simulink model "Control_try_final_2020b"  (R2020b)
settings: Solver=VariableStepAuto  StartTime=0.0  StopTime=inf  RelTol=1e-3
undefined symbols (not defined in the file or in its folder): DiscIntNeverNeededParam
libraries: mobileRoboticsLib x25
(part 5 of 7)

== system Control_try_final_2020b/Team_1_behaviour/T1R3 (defender 1)/Team 1 Behaviour1/min_Distance_Finder/Distance1 ==
  R_1_loc : Inport
  R_3_loc : Inport  Port=2
  Demux : Demux  Outputs=3
  Demux1 : Demux  Outputs=3
  Square : Math  Operator=square  SaturateOnIntegerOverflow=on
  Square Root : Sqrt  SaturateOnIntegerOverflow=on
  Square1 : Math  Operator=square  SaturateOnIntegerOverflow=on
  Sum : Sum  Inputs=|+-
  Sum1 : Sum  Inputs=|+-
  Sum2 : Sum  Inputs=|++
  R1_R3_dis : Outport
  wires:
  Square1/1 -> Sum2/2
  Demux/2 -> Sum1/1
  Sum2/1 -> Square Root/1
  Square/1 -> Sum2/1
  Demux/1 -> Sum/1
  Sum1/1 -> Square1/1
  Demux1/2 -> Sum1/2
  Sum/1 -> Square/1
  Demux1/1 -> Sum/2
  R_1_loc/1 -> Demux/1
  R_3_loc/1 -> Demux1/1
  Square Root/1 -> R1_R3_dis/1

== system Control_try_final_2020b/Team_1_behaviour/T1R3 (defender 1)/Team 1 Behaviour1/min_Distance_Finder/Distance2 ==
  R_1_loc : Inport
  R_4_loc : Inport  Port=2
  Demux : Demux  Outputs=3
  Demux1 : Demux  Outputs=3
  Square : Math  Operator=square  SaturateOnIntegerOverflow=on
  Square Root : Sqrt  SaturateOnIntegerOverflow=on
  Square1 : Math  Operator=square  SaturateOnIntegerOverflow=on
  Sum : Sum  Inputs=|+-
  Sum1 : Sum  Inputs=|+-
  Sum2 : Sum  Inputs=|++
  R1_R4_dis : Outport
  wires:
  Square1/1 -> Sum2/2
  Demux/2 -> Sum1/1
  Sum2/1 -> Square Root/1
  Square/1 -> Sum2/1
  Demux/1 -> Sum/1
  Sum1/1 -> Square1/1
  Demux1/2 -> Sum1/2
  Sum/1 -> Square/1
  Demux1/1 -> Sum/2
  R_1_loc/1 -> Demux/1
  R_4_loc/1 -> Demux1/1
  Square Root/1 -> R1_R4_dis/1

== system Control_try_final_2020b/Team_1_behaviour/T1R3 (defender 1)/Team 1 Behaviour1/min_Distance_Finder/R2_O_dist_val ==
  R_1_loc : Inport
  R_2_loc : Inport  Port=2
  sen_1_val : Inport  Port=3
  Chart : Stateflow chart  TreatAsAtomicUnit=on
  y : Outport
  wires:
  sen_1_val/1 -> Chart/2(sen_1_val)
  R_1_loc/1 -> Chart/1(R_1_loc)
  R_2_loc/1 -> Chart/3(R_2_loc)
  Chart/1(dist) -> y/1

== system Control_try_final_2020b/Team_1_behaviour/T1R3 (defender 1)/Team 1 Behaviour1/min_Distance_Finder/R3_O_dist_val ==
  R_1_loc : Inport
  R_2_loc : Inport  Port=2
  sen_1_val : Inport  Port=3
  Chart : Stateflow chart  TreatAsAtomicUnit=on
  y : Outport
  wires:
  Chart/1(dist) -> y/1
  R_2_loc/1 -> Chart/3(R_2_loc)
  R_1_loc/1 -> Chart/1(R_1_loc)
  sen_1_val/1 -> Chart/2(sen_1_val)

== system Control_try_final_2020b/Team_1_behaviour/T1R3 (defender 1)/Team 1 Behaviour1/min_Distance_Finder/R4_O_dist_val ==
  R_1_loc : Inport
  R_2_loc : Inport  Port=2
  sen_1_val : Inport  Port=3
  Chart : Stateflow chart  TreatAsAtomicUnit=on
  y : Outport
  wires:
  sen_1_val/1 -> Chart/2(sen_1_val)
  R_1_loc/1 -> Chart/1(R_1_loc)
  R_2_loc/1 -> Chart/3(R_2_loc)
  Chart/1(dist) -> y/1

== system Control_try_final_2020b/Team_2_Behaviour/T2_R2(defender)/Team 1 Behaviour1/Subsystem/If Action Subsystem ==
  In1 : Inport
  Action Port : ActionPort  ActionPortLabel=if(u1 > 0)
  Out1 : Outport
  wires:
  In1/1 -> Out1/1

== system Control_try_final_2020b/Team_2_Behaviour/T2_R2(defender)/Team 1 Behaviour1/Subsystem/If Action Subsystem1 ==
  In1 : Inport
  Action Port : ActionPort  ActionPortLabel=else
  Out1 : Outport
  wires:
  In1/1 -> Out1/1

== system Control_try_final_2020b/Team_2_Behaviour/T2_R2(defender)/Team 1 Behaviour1/Subsystem1/If Action Subsystem ==
  In1 : Inport
  Action Port : ActionPort  ActionPortLabel=if(u1 < 5.5)
  reset_pos : Outport
  wires:
  In1/1 -> reset_pos/1

== system Control_try_final_2020b/Team_2_Behaviour/T2_R2(defender)/Team 1 Behaviour1/Subsystem1/If Action Subsystem1 ==
  In1 : Inport
  Action Port : ActionPort  ActionPortLabel=else
  reset_pos : Outport
  wires:
  In1/1 -> reset_pos/1

== system Control_try_final_2020b/Team_2_Behaviour/T2_R2(defender)/Team 1 Behaviour1/Subsystem2/If Action Subsystem ==
  In1 : Inport
  Action Port : ActionPort  ActionPortLabel=if(u1 < 5.5)
  reset_pos : Outport
  wires:
  In1/1 -> reset_pos/1

== system Control_try_final_2020b/Team_2_Behaviour/T2_R2(defender)/Team 1 Behaviour1/Subsystem2/If Action Subsystem1 ==
  In1 : Inport
  Action Port : ActionPort  ActionPortLabel=else
  reset_pos : Outport
  wires:
  In1/1 -> reset_pos/1

== system Control_try_final_2020b/Team_2_Behaviour/T2_R2(defender)/Team 1 Behaviour1/kick_direction1/Angle Finder1 ==
  In1 : Inport
  Abs : Abs
  Atan : Trigonometry  Operator=atan
  Demux : Demux  Outputs=2
  Divide : Product  Inputs=/*
  angle : Outport
  wires:
  Divide/1 -> Atan/1
  Demux/2 -> Divide/2
  Demux/1 -> Divide/1
  Atan/1 -> Abs/1
  Abs/1 -> angle/1
  In1/1 -> Demux/1

== system Control_try_final_2020b/Team_2_Behaviour/T2_R2(defender)/Team 1 Behaviour1/min_Distance_Finder/Distance1 ==
  R_1_loc : Inport
  R_3_loc : Inport  Port=2
  Demux : Demux  Outputs=3
  Demux1 : Demux  Outputs=3
  Square : Math  Operator=square  SaturateOnIntegerOverflow=on
  Square Root : Sqrt  SaturateOnIntegerOverflow=on
  Square1 : Math  Operator=square  SaturateOnIntegerOverflow=on
  Sum : Sum  Inputs=|+-
  Sum1 : Sum  Inputs=|+-
  Sum2 : Sum  Inputs=|++
  R1_R3_dis : Outport
  wires:
  Square1/1 -> Sum2/2
  Demux/2 -> Sum1/1
  Sum2/1 -> Square Root/1
  Square/1 -> Sum2/1
  Demux/1 -> Sum/1
  Sum1/1 -> Square1/1
  Demux1/2 -> Sum1/2
  Sum/1 -> Square/1
  Demux1/1 -> Sum/2
  R_1_loc/1 -> Demux/1
  R_3_loc/1 -> Demux1/1
  Square Root/1 -> R1_R3_dis/1

== system Control_try_final_2020b/Team_2_Behaviour/T2_R2(defender)/Team 1 Behaviour1/min_Distance_Finder/Distance2 ==
  R_1_loc : Inport
  R_4_loc : Inport  Port=2
  Demux : Demux  Outputs=3
  Demux1 : Demux  Outputs=3
  Square : Math  Operator=square  SaturateOnIntegerOverflow=on
  Square Root : Sqrt  SaturateOnIntegerOverflow=on
  Square1 : Math  Operator=square  SaturateOnIntegerOverflow=on
  Sum : Sum  Inputs=|+-
  Sum1 : Sum  Inputs=|+-
  Sum2 : Sum  Inputs=|++
  R1_R4_dis : Outport
  wires:
  Square1/1 -> Sum2/2
  Demux/2 -> Sum1/1
  Sum2/1 -> Square Root/1
  Square/1 -> Sum2/1
  Demux/1 -> Sum/1
  Sum1/1 -> Square1/1
  Demux1/2 -> Sum1/2
  Sum/1 -> Square/1
  Demux1/1 -> Sum/2
  R_1_loc/1 -> Demux/1
  R_4_loc/1 -> Demux1/1
  Square Root/1 -> R1_R4_dis/1

== system Control_try_final_2020b/Team_2_Behaviour/T2_R2(defender)/Team 1 Behaviour1/min_Distance_Finder/R2_O_dist_val ==
  R_1_loc : Inport
  R_2_loc : Inport  Port=2
  sen_1_val : Inport  Port=3
  Chart : Stateflow chart  TreatAsAtomicUnit=on
  y : Outport
  wires:
  sen_1_val/1 -> Chart/2(sen_1_val)
  R_1_loc/1 -> Chart/1(R_1_loc)
  R_2_loc/1 -> Chart/3(R_2_loc)
  Chart/1(dist) -> y/1

== system Control_try_final_2020b/Team_2_Behaviour/T2_R2(defender)/Team 1 Behaviour1/min_Distance_Finder/R3_O_dist_val ==
  R_1_loc : Inport
  R_2_loc : Inport  Port=2
  sen_1_val : Inport  Port=3
  Chart : Stateflow chart  TreatAsAtomicUnit=on
  y : Outport
  wires:
  Chart/1(dist) -> y/1
  R_2_loc/1 -> Chart/3(R_2_loc)
  R_1_loc/1 -> Chart/1(R_1_loc)
  sen_1_val/1 -> Chart/2(sen_1_val)

== system Control_try_final_2020b/Team_2_Behaviour/T2_R2(defender)/Team 1 Behaviour1/min_Distance_Finder/R4_O_dist_val ==
  R_1_loc : Inport
  R_2_loc : Inport  Port=2
  sen_1_val : Inport  Port=3
  Chart : Stateflow chart  TreatAsAtomicUnit=on
  y : Outport
  wires:
  sen_1_val/1 -> Chart/2(sen_1_val)
  R_1_loc/1 -> Chart/1(R_1_loc)
  R_2_loc/1 -> Chart/3(R_2_loc)
  Chart/1(dist) -> y/1

== system Control_try_final_2020b/Team_2_Behaviour/T2_R2(defender)/Team 1 Behaviour1/min_Distance_Finder/nearest robot distance ==
  R_1_loc : Inport
  sen_1_val : Inport  Port=2
  Chart : Stateflow chart  TreatAsAtomicUnit=on
  y : Outport
  wires:
  Chart/1(dist) -> y/1
  R_1_loc/1 -> Chart/1(R_1_loc)
  sen_1_val/1 -> Chart/2(sen_1_val)

== system Control_try_final_2020b/Team_2_Behaviour/T2_R3(Attacker 1)/Team 1 Behaviour1/Subsystem/If Action Subsystem ==
  In1 : Inport
  Action Port : ActionPort  ActionPortLabel=if(u1 > 0)
  Out1 : Outport
  wires:
  In1/1 -> Out1/1

== system Control_try_final_2020b/Team_2_Behaviour/T2_R3(Attacker 1)/Team 1 Behaviour1/Subsystem/If Action Subsystem1 ==
  In1 : Inport
  Action Port : ActionPort  ActionPortLabel=else
  Out1 : Outport
  wires:
  In1/1 -> Out1/1

== system Control_try_final_2020b/Team_2_Behaviour/T2_R3(Attacker 1)/Team 1 Behaviour1/Subsystem1/If Action Subsystem ==
  In1 : Inport
  Action Port : ActionPort  ActionPortLabel=if(u1 > 5.5)
  reset_pos : Outport
  wires:
  In1/1 -> reset_pos/1

== system Control_try_final_2020b/Team_2_Behaviour/T2_R3(Attacker 1)/Team 1 Behaviour1/Subsystem1/If Action Subsystem1 ==
  In1 : Inport
  Action Port : ActionPort  ActionPortLabel=else
  reset_pos : Outport
  wires:
  In1/1 -> reset_pos/1

== system Control_try_final_2020b/Team_2_Behaviour/T2_R3(Attacker 1)/Team 1 Behaviour1/kick_direction1/Angle Finder1 ==
  In1 : Inport
  Abs : Abs
  Atan : Trigonometry  Operator=atan
  Demux : Demux  Outputs=2
  Divide : Product  Inputs=/*
  angle : Outport
  wires:
  Divide/1 -> Atan/1
  Demux/2 -> Divide/2
  Demux/1 -> Divide/1
  Atan/1 -> Abs/1
  Abs/1 -> angle/1
  In1/1 -> Demux/1

== system Control_try_final_2020b/Team_2_Behaviour/T2_R3(Attacker 1)/Team 1 Behaviour1/min_Distance_Finder1/Distance1 ==
  R_1_loc : Inport
  R_3_loc : Inport  Port=2
  Demux : Demux  Outputs=3
  Demux1 : Demux  Outputs=3
  Square : Math  Operator=square  SaturateOnIntegerOverflow=on
  Square Root : Sqrt  SaturateOnIntegerOverflow=on
  Square1 : Math  Operator=square  SaturateOnIntegerOverflow=on
  Sum : Sum  Inputs=|+-
  Sum1 : Sum  Inputs=|+-
  Sum2 : Sum  Inputs=|++
  R1_R3_dis : Outport
  wires:
  Square1/1 -> Sum2/2
  Demux/2 -> Sum1/1
  Sum2/1 -> Square Root/1
  Square/1 -> Sum2/1
  Demux/1 -> Sum/1
  Sum1/1 -> Square1/1
  Demux1/2 -> Sum1/2
  Sum/1 -> Square/1
  Demux1/1 -> Sum/2
  R_1_loc/1 -> Demux/1
  R_3_loc/1 -> Demux1/1
  Square Root/1 -> R1_R3_dis/1

== system Control_try_final_2020b/Team_2_Behaviour/T2_R3(Attacker 1)/Team 1 Behaviour1/min_Distance_Finder1/Distance2 ==
  R_1_loc : Inport
  R_4_loc : Inport  Port=2
  Demux : Demux  Outputs=3
  Demux1 : Demux  Outputs=3
  Square : Math  Operator=square  SaturateOnIntegerOverflow=on
  Square Root : Sqrt  SaturateOnIntegerOverflow=on
  Square1 : Math  Operator=square  SaturateOnIntegerOverflow=on
  Sum : Sum  Inputs=|+-
  Sum1 : Sum  Inputs=|+-
  Sum2 : Sum  Inputs=|++
  R1_R4_dis : Outport
  wires:
  Square1/1 -> Sum2/2
  Demux/2 -> Sum1/1
  Sum2/1 -> Square Root/1
  Square/1 -> Sum2/1
  Demux/1 -> Sum/1
  Sum1/1 -> Square1/1
  Demux1/2 -> Sum1/2
  Sum/1 -> Square/1
  Demux1/1 -> Sum/2
  R_1_loc/1 -> Demux/1
  R_4_loc/1 -> Demux1/1
  Square Root/1 -> R1_R4_dis/1

== system Control_try_final_2020b/Team_2_Behaviour/T2_R3(Attacker 1)/Team 1 Behaviour1/min_Distance_Finder1/R2_O_dist_val ==
  R_1_loc : Inport
  R_2_loc : Inport  Port=2
  sen_1_val : Inport  Port=3
  Chart : Stateflow chart  TreatAsAtomicUnit=on
  y : Outport
  wires:
  sen_1_val/1 -> Chart/2(sen_1_val)
  R_1_loc/1 -> Chart/1(R_1_loc)
  R_2_loc/1 -> Chart/3(R_2_loc)
  Chart/1(dist) -> y/1

== system Control_try_final_2020b/Team_2_Behaviour/T2_R3(Attacker 1)/Team 1 Behaviour1/min_Distance_Finder1/R3_O_dist_val ==
  R_1_loc : Inport
  R_2_loc : Inport  Port=2
  sen_1_val : Inport  Port=3
  Chart : Stateflow chart  TreatAsAtomicUnit=on
  y : Outport
  wires:
  Chart/1(dist) -> y/1
  R_2_loc/1 -> Chart/3(R_2_loc)
  R_1_loc/1 -> Chart/1(R_1_loc)
  sen_1_val/1 -> Chart/2(sen_1_val)

== system Control_try_final_2020b/Team_2_Behaviour/T2_R3(Attacker 1)/Team 1 Behaviour1/min_Distance_Finder1/R4_O_dist_val ==
  R_1_loc : Inport
  R_2_loc : Inport  Port=2
  sen_1_val : Inport  Port=3
  Chart : Stateflow chart  TreatAsAtomicUnit=on
  y : Outport
  wires:
  sen_1_val/1 -> Chart/2(sen_1_val)
  R_1_loc/1 -> Chart/1(R_1_loc)
  R_2_loc/1 -> Chart/3(R_2_loc)
  Chart/1(dist) -> y/1

== system Control_try_final_2020b/Team_2_Behaviour/T2_R3(Attacker 1)/Team 1 Behaviour1/min_Distance_Finder1/nearest robot distance ==
  R_1_loc : Inport
  sen_1_val : Inport  Port=2
  Chart : Stateflow chart  TreatAsAtomicUnit=on
  y : Outport
  wires:
  Chart/1(dist) -> y/1
  R_1_loc/1 -> Chart/1(R_1_loc)
  sen_1_val/1 -> Chart/2(sen_1_val)

== system Control_try_final_2020b/Team_2_Behaviour/T3_R4(Attacker 2)/Team 1 Behaviour1/Subsystem3/If Action Subsystem ==
  In1 : Inport
  Action Port : ActionPort  ActionPortLabel=if(u1 > 0)
  Out1 : Outport
  wires:
  In1/1 -> Out1/1

== system Control_try_final_2020b/Team_2_Behaviour/T3_R4(Attacker 2)/Team 1 Behaviour1/Subsystem3/If Action Subsystem1 ==
  In1 : Inport
  Action Port : ActionPort  ActionPortLabel=else
  Out1 : Outport
  wires:
  In1/1 -> Out1/1

== system Control_try_final_2020b/Team_2_Behaviour/T3_R4(Attacker 2)/Team 1 Behaviour1/Subsystem4/If Action Subsystem ==
  In1 : Inport
  Action Port : ActionPort  ActionPortLabel=if(u1 > 5.5)
  reset_pos : Outport
  wires:
  In1/1 -> reset_pos/1

== system Control_try_final_2020b/Team_2_Behaviour/T3_R4(Attacker 2)/Team 1 Behaviour1/Subsystem4/If Action Subsystem1 ==
  In1 : Inport
  Action Port : ActionPort  ActionPortLabel=else
  reset_pos : Outport
  wires:
  In1/1 -> reset_pos/1

== system Control_try_final_2020b/Team_2_Behaviour/T3_R4(Attacker 2)/Team 1 Behaviour1/kick_direction2/Angle Finder1 ==
  In1 : Inport
  Abs : Abs
  Atan : Trigonometry  Operator=atan
  Demux : Demux  Outputs=2
  Divide : Product  Inputs=/*
  angle : Outport
  wires:
  Divide/1 -> Atan/1
  Demux/2 -> Divide/2
  Demux/1 -> Divide/1
  Atan/1 -> Abs/1
  Abs/1 -> angle/1
  In1/1 -> Demux/1

== system Control_try_final_2020b/Team_2_Behaviour/T3_R4(Attacker 2)/Team 1 Behaviour1/min_Distance_Finder1/Distance1 ==
  R_1_loc : Inport
  R_3_loc : Inport  Port=2
  Demux : Demux  Outputs=3
  Demux1 : Demux  Outputs=3
  Square : Math  Operator=square  SaturateOnIntegerOverflow=on
  Square Root : Sqrt  SaturateOnIntegerOverflow=on
  Square1 : Math  Operator=square  SaturateOnIntegerOverflow=on
  Sum : Sum  Inputs=|+-
  Sum1 : Sum  Inputs=|+-
  Sum2 : Sum  Inputs=|++
  R1_R3_dis : Outport
  wires:
  Square1/1 -> Sum2/2
  Demux/2 -> Sum1/1
  Sum2/1 -> Square Root/1
  Square/1 -> Sum2/1
  Demux/1 -> Sum/1
  Sum1/1 -> Square1/1
  Demux1/2 -> Sum1/2
  Sum/1 -> Square/1
  Demux1/1 -> Sum/2
  R_1_loc/1 -> Demux/1
  R_3_loc/1 -> Demux1/1
  Square Root/1 -> R1_R3_dis/1

== system Control_try_final_2020b/Team_2_Behaviour/T3_R4(Attacker 2)/Team 1 Behaviour1/min_Distance_Finder1/Distance2 ==
  R_1_loc : Inport
  R_4_loc : Inport  Port=2
  Demux : Demux  Outputs=3
  Demux1 : Demux  Outputs=3
  Square : Math  Operator=square  SaturateOnIntegerOverflow=on
  Square Root : Sqrt  SaturateOnIntegerOverflow=on
  Square1 : Math  Operator=square  SaturateOnIntegerOverflow=on
  Sum : Sum  Inputs=|+-
  Sum1 : Sum  Inputs=|+-
  Sum2 : Sum  Inputs=|++
  R1_R4_dis : Outport
  wires:
  Square1/1 -> Sum2/2
  Demux/2 -> Sum1/1
  Sum2/1 -> Square Root/1
  Square/1 -> Sum2/1
  Demux/1 -> Sum/1
  Sum1/1 -> Square1/1
  Demux1/2 -> Sum1/2
  Sum/1 -> Square/1
  Demux1/1 -> Sum/2
  R_1_loc/1 -> Demux/1
  R_4_loc/1 -> Demux1/1
  Square Root/1 -> R1_R4_dis/1

== system Control_try_final_2020b/Team_2_Behaviour/T3_R4(Attacker 2)/Team 1 Behaviour1/min_Distance_Finder1/R2_O_dist_val ==
  R_1_loc : Inport
  R_2_loc : Inport  Port=2
  sen_1_val : Inport  Port=3
  Chart : Stateflow chart  TreatAsAtomicUnit=on
  y : Outport
  wires:
  sen_1_val/1 -> Chart/2(sen_1_val)
  R_1_loc/1 -> Chart/1(R_1_loc)
  R_2_loc/1 -> Chart/3(R_2_loc)
  Chart/1(dist) -> y/1

== system Control_try_final_2020b/Team_2_Behaviour/T3_R4(Attacker 2)/Team 1 Behaviour1/min_Distance_Finder1/R3_O_dist_val ==
  R_1_loc : Inport
  R_2_loc : Inport  Port=2
  sen_1_val : Inport  Port=3
  Chart : Stateflow chart  TreatAsAtomicUnit=on
  y : Outport
  wires:
  Chart/1(dist) -> y/1
  R_2_loc/1 -> Chart/3(R_2_loc)
  R_1_loc/1 -> Chart/1(R_1_loc)
  sen_1_val/1 -> Chart/2(sen_1_val)

== system Control_try_final_2020b/Team_2_Behaviour/T3_R4(Attacker 2)/Team 1 Behaviour1/min_Distance_Finder1/R4_O_dist_val ==
  R_1_loc : Inport
  R_2_loc : Inport  Port=2
  sen_1_val : Inport  Port=3
  Chart : Stateflow chart  TreatAsAtomicUnit=on
  y : Outport
  wires:
  sen_1_val/1 -> Chart/2(sen_1_val)
  R_1_loc/1 -> Chart/1(R_1_loc)
  R_2_loc/1 -> Chart/3(R_2_loc)
  Chart/1(dist) -> y/1

== system Control_try_final_2020b/Team_2_Behaviour/T3_R4(Attacker 2)/Team 1 Behaviour1/min_Distance_Finder1/nearest robot distance ==
  R_1_loc : Inport
  sen_1_val : Inport  Port=2
  Chart : Stateflow chart  TreatAsAtomicUnit=on
  y : Outport
  wires:
  Chart/1(dist) -> y/1
  R_1_loc/1 -> Chart/1(R_1_loc)
  sen_1_val/1 -> Chart/2(sen_1_val)

== matlab function Control_try_final_2020b/Team_1_behaviour/T1R3 (defender 1)/Team 1 Behaviour1/min_Distance_Finder/zero_padding ==
  data: u input; y output
function y = pad(u)
% Zero-pads object detections to work with arrays of buses

y = zeros(7,3);
numElems = min(size(u,1),7);
for idx = 1:numElems
   y(idx,1:3) = u(idx,1:3); 
end
end

== stateflow chart Control_try_final_2020b/Enviornment/Chart1 ==
  state P1_kick
    du:
    KF = [p1(1);p1(2);p1(3);p1(4)]
    bot_tag = 1
  state P5_kick
    du:
    KF = [p5(1);p5(2);p5(3);p5(4)]
    bot_tag = 5
  state no_ball_kick
    du:
    KF = [0;0;0;0]
  state P2_kick
    du:
    KF = p2
    bot_tag = 2
  state P6_kick
    du:
    KF = p6
    bot_tag = 6
  state P3_kick
    du:
    KF = p3
    bot_tag = 3
  state P7_kick
    du:
    KF = p7
    bot_tag = 7
  state P4_kick
    du:
    KF = p4
    bot_tag = 4
  state P8_kick
    du:
    KF = p8
    bot_tag = 8
  (default) -> no_ball_kick
  P5_kick -> no_ball_kick : [p5(4) == 0]
  P1_kick -> no_ball_kick : [p1(4) == 0]
  no_ball_kick -> P5_kick [order 5] : [p5(4) == 1]
  no_ball_kick -> P1_kick [order 1] : [p1(4) == 1]
  no_ball_kick -> P2_kick [order 2] : [p2(4) == 1]
  no_ball_kick -> P6_kick [order 6] : [p6(4) == 1]
  P2_kick -> no_ball_kick : [p2(4) == 0]
  P6_kick -> no_ball_kick : [p6(4) == 0]
  P3_kick -> no_ball_kick : [p3(4) == 0]
  P7_kick -> no_ball_kick : [p7(4) == 0]
  no_ball_kick -> P7_kick [order 7] : [p7(4) == 1]
  no_ball_kick -> P3_kick [order 3] : [p3(4) == 1]
  no_ball_kick -> P8_kick [order 8] : [p8(4) == 1]
  no_ball_kick -> P4_kick [order 4] : [p4(4) == 1]
  P4_kick -> no_ball_kick : [p4(4) == 0]
  P8_kick -> no_ball_kick : [p8(4) == 0]
  data: bot_tag output; p1 input; p2 input; p3 input; p4 input; p5 input; p6 input; p7 input; p8 input; KF output

== stateflow chart Control_try_final_2020b/Team_1_behaviour/T1R1(Goal_Keeper)/Ball_in_D/Chart ==
  state second_coordinate
    du:
    actual_angle = -pi +angle + angle_bot;
  state first_coordinate
    du:
    actual_angle = angle_bot - angle;
  state ffourth_coordinate
    du:
    actual_angle = -(2*pi) + angle + angle_bot
  state Third_coordinate
    du:
    actual_angle =-(pi) - angle + angle_bot;
  (default) -> first_coordinate
  first_coordinate -> second_coordinate [order 1] : [ Rx>Bx && Ry<By ]
  second_coordinate -> first_coordinate [order 1] : [ Rx<Bx && Ry<By]
  ffourth_coordinate -> second_coordinate [order 1] : [ Rx>Bx && Ry<By ]
  first_coordinate -> Third_coordinate [order 3] : [ Rx>Bx && Ry>By]
  second_coordinate -> Third_coordinate [order 3] : [ Rx>Bx && Ry>By ]
  Third_coordinate -> second_coordinate [order 1] : [ Rx>Bx && Ry<By ]
  second_coordinate -> ffourth_coordinate [order 2] : [ Rx<Bx && Ry>By ]
  Third_coordinate -> first_coordinate [order 2] : [ Rx<Bx && Ry<By ]
  ffourth_coordinate -> first_coordinate [order 2] : [ Rx<Bx && Ry<By ]
  first_coordinate -> ffourth_coordinate [order 2] : [ Rx<Bx && Ry>By ]
  Third_coordinate -> ffourth_coordinate [order 3] : [ Rx<Bx && Ry>By ]
  ffourth_coordinate -> Third_coordinate [order 3] : [ Rx>Bx && Ry>By]
  data: Bx input; By input; Rx input; Ry input; angle input; actual_angle output; angle_bot input

== stateflow chart Control_try_final_2020b/Team_1_behaviour/T1R1(Goal_Keeper)/Ball_in_D/Chart3 ==
  state stop
    du:
    w = 0;
    v=0.25 * velocity;
  state RCW
    du:
    w = -1*1;
    v=0;
  state RCCW
    du:
    w =1*1;
    v=0;
  (default) -> stop
  stop -> RCCW [order 2] : [after(1,sec) && DT > 0]
  stop -> RCW [order 1] : [after(1,sec) && DT < 0]
  RCW -> stop [order 1] : [DT<= 0.1 && DT>= -0.1]
  RCCW -> stop [order 1] : [DT<= 0.1 && DT>= -0.1]
  RCCW -> RCW [order 2] : [DT>0]
  RCW -> RCCW [order 2] : [DT<0]
  data: velocity input; v output; DT input; w output

== stateflow chart Control_try_final_2020b/Team_1_behaviour/T1R1(Goal_Keeper)/Ball_in_D/Velocity_Decider ==
  state Robot_Far
    du:
    velocity = 1;
    kick = 0;
  state Robot_Close
    du:
    velocity = 0;
    kick = 1;
  (default) -> Robot_Far
  Robot_Far -> Robot_Close : [DBR <= 0.25]
  Robot_Close -> Robot_Far : [DBR > 0.25]
  data: kick output; DBR input; velocity output

== stateflow chart Control_try_final_2020b/Team_2_Behaviour/T2_R3(Attacker 1)/Team 1 Behaviour1/Chart4 ==
  state go_to_ball
    du:
    kick = 0;
    pass_beh = 0;
    if(distance_to_ball < 0.25)
    pass_beh = pass_behaviour_controller(distance_to_goal,nearest_op,nearest_team);
    i = 0;
    else
    velocity = 0.44;
    end
  state avoid
    velocity = -0.44;
  state pass
    du:
    velocity = 0;
    kick = 1;
  state shoot
    du:
    velocity = 0;
    kick = 1;
  state dribble
    du:
    velocity = 0;
    kick = 1;
  (default) -> go_to_ball
  go_to_ball -> avoid [order 4] : [nearest_rob < 0.3 && nearest_rob < 0 ]
  avoid -> go_to_ball : [nearest_rob > 1 || nearest_rob == 0]
  go_to_ball -> pass [order 1] : [pass_beh == 1&& distance_to_ball < 0.25 ]
  dribble -> go_to_ball : [kick == 1]
  go_to_ball -> dribble [order 3] : [pass_beh == 2 && distance_to_ball < 0.25 ]
  pass -> go_to_ball : [kick == 1]
  go_to_ball -> shoot [order 2] : [pass_beh == 3 && distance_to_ball < 0.25 ]
  shoot -> go_to_ball : [kick == 1]
  data: distancetogoal function_input; nearest_oponent_distance function_input; nearest_team_player_distance function_input; pass_behaviour function_output; kick output =0; distance_to_ball input; velocity output; nearest_team input; nearest_op input; distance_to_goal input; pass_beh output =0; i local =1; nearest_rob input
  function pass_behaviour  = pass_behaviour_controller(distancetogoal,nearest_oponent_distance,nearest_team_player_distance):
    | function pass_behaviour  = pass_behaviour_controller(distancetogoal,nearest_oponent_distance,nearest_team_player_distance)
    | %PASS_BEHAVIOR Summary of this function goes here
    | %   Detailed explanation goes here
    | behaviourFuzzyFile= getFISCodeGenerationData('pass_behaviour.fis');
    | b = evalfis(behaviourFuzzyFile,[distancetogoal,nearest_oponent_distance,nearest_team_player_distance]);
    | 
    | if ( b<0.4 )
    | pass_behaviour=1;
    | elseif ( 0.4<=b && b<0.6 )
    | pass_behaviour=2;
    | else
    | pass_behaviour=3;
    | end
    | 
    | end

== stateflow chart Control_try_final_2020b/Team_1_behaviour/T1R1(Goal_Keeper)/Ball_in_D/kick_direction/Chart1 ==
  state x_pos
    du:
    Vx = 1
  state x_neg
    du:
    Vx = -1
  (default) -> x_pos
  x_pos -> x_neg : [x > 0]
  x_neg -> x_pos : [x<1]
  data: Vx output; x input

== stateflow chart Control_try_final_2020b/Team_1_behaviour/T1R1(Goal_Keeper)/Ball_in_D/kick_direction/Chart2 ==
  state y_pos
    du:
    Vy = 1
  state y_neg
    du:
    Vy = -1
  (default) -> y_pos
  y_pos -> y_neg : [y > 0]
  y_neg -> y_pos : [y<1]
  data: y input; Vy output

== stateflow chart Control_try_final_2020b/Team_1_behaviour/T1R3 (Defender 2)/Chart ==
  state reaching_foul
    du:
    velocity_UA = 1;
    dest = [bx;by;0];
  state ball_in_other_half_did_foul
    en:
    if (foul_loc_y>=7)
    dest = [foul_loc_x;foul_loc_y - 1;0];
    elseif(foul_loc_y<=1)
    dest = [foul_loc_x;foul_loc_y + 1;0];
    end
    kick_UA = 1;
    stop = 1;
  state throwing_foul_not_done
    du:
    dest = [bx;by;0];
    kick_UA = 0;
  state ball_in_our_half
    en:
    dest = [5;4;0];
    kick_UA = 1;
  state stop_bot1
    du:
    velocity_UA = 1;
    dest = [bx;by;0];
  state dont_stop_bot1
    du:
    velocity_UA = 1;
    dest = [bx;by;0];
  state throwing_foul_done
    du:
  state init_pos_reached2
    du:
    velocity_UA = 1;
    dest = [bx;by;0];
  state in_play1
    du:
    dest = [bx;by;0];
    kick_UA = 0;
    stop = 0
    velocity_UA = 0;
  state goal1
    en:
    dest = [5;4;0];
    kick_UA = 1;
    if (did_goal == 1)
    stop = 1;
    else
    stop = 0;
    end
  state init_pos_reached1
    du:
  throwing_foul_not_done -> ball_in_our_half [order 2] : [foul_loc_x < 5.5]
  ball_in_other_half_did_foul -> reaching_foul : [R_2_loc(1) < foul_loc_x + 0.25 &&  R_2_loc(1) > foul_loc_x- 0.25 && R_2_loc(2) < foul_loc_y + 1.25 &&  R_2_loc(2) > foul_loc_y - 1.25 && after(3,sec)]
  init_pos_reached1 -> dont_stop_bot1 [order 2] : [stop == 0]
  reaching_foul -> in_play1 : [bx >foul_loc_x + 0.1  || bx < foul_loc_x - 0.1|| by >foul_loc_y + 0.1 || by<foul_loc_y - 0.1]
  throwing_foul_done -> ball_in_other_half_did_foul [order 1] : [foul_loc_x > 5.5]
  in_play1 -> throwing_foul_not_done [order 3] : [foul_team_right == 1]
  throwing_foul_not_done -> in_play1 [order 1] : [foul_loc_x > 5.5 && after(2,sec)]
  init_pos_reached1 -> stop_bot1 [order 1] : [stop == 1]
  throwing_foul_done -> ball_in_our_half [order 2] : [foul_loc_x < 5.5]
  ball_in_our_half -> init_pos_reached2 : [R_2_loc(1) <5.25 &&  R_2_loc(1) >4.75 && R_2_loc(2) <4.25 &&  R_2_loc(2) >3.75 && after(2,sec)]
  in_play1 -> throwing_foul_done [order 2] : [foul_team_left == 1]
  dont_stop_bot1 -> in_play1 : [reset == 0 && after(3,sec)]
  stop_bot1 -> in_play1 : [bx > 5.6 || bx < 5.4 || by >4.1 || by<3.9]
  (default) -> in_play1
  init_pos_reached2 -> in_play1 : [[bx >foul_loc_x + 0.1  || bx < foul_loc_x - 0.1|| by >foul_loc_y + 0.1 || by<foul_loc_y - 0.1]]
  goal1 -> init_pos_reached1 : [R_2_loc(1) <5.25 &&  R_2_loc(1) >4.75 && R_2_loc(2) <4.25 &&  R_2_loc(2) >3.75 && after(3,sec) ]
  in_play1 -> goal1 [order 1] : [reset == 1]
  data: R_2_loc input; bx input; by input; foul_team_right input; foul_team_left input; did_goal input; foul_loc_x input; foul_loc_y input; reset input; dest output; kick_UA output; velocity_UA output; stop local

== stateflow chart Control_try_final_2020b/Team_2_Behaviour/T2_R2(defender)/Chart ==
  state reaching_foul
    du:
    velocity_UA = 1;
    dest = [bx;by;0];
  state ball_in_other_half_did_foul
    en:
    if (foul_loc_y>=7)
    dest = [foul_loc_x;foul_loc_y - 1;0];
    elseif(foul_loc_y<=1)
    dest = [foul_loc_x;foul_loc_y + 1;0];
    end
    kick_UA = 1;
    stop = 1;
  state throwing_foul_done
    du:
  state throwing_foul_not_done
    du:
    dest = [bx;by;0];
    kick_UA = 0;
  state ball_in_our_half
    en:
    dest = [7.25;2.5;0];
    kick_UA = 1;
  state stop_bot1
    du:
    velocity_UA = 1;
    dest = [bx;by;0];
  state dont_stop_bot1
    du:
    velocity_UA = 1;
    dest = [bx;by;0];
  state init_pos_reached2
    du:
    velocity_UA = 1;
    dest = [bx;by;0];
  state in_play1
    du:
    dest = [bx;by;0];
    kick_UA = 0;
    stop = 0
    velocity_UA = 0;
  state goal1
    en:
    dest = [7.25;2.5;0];
    kick_UA = 1;
    if (did_goal == 1)
    stop = 1;
    else
    stop = 0;
    end
  state init_pos_reached1
    du:
  throwing_foul_not_done -> ball_in_our_half [order 2] : [foul_loc_x < 6]
  ball_in_other_half_did_foul -> reaching_foul : [R_2_loc(1) < foul_loc_x + 0.25 &&  R_2_loc(1) > foul_loc_x- 0.25 && R_2_loc(2) < foul_loc_y + 1.25 &&  R_2_loc(2) > foul_loc_y - 1.25 && after(3,sec)]
  reaching_foul -> in_play1 : [bx >foul_loc_x + 0.1  || bx < foul_loc_x - 0.1|| by >foul_loc_y + 0.1 || by<foul_loc_y - 0.1]
  throwing_foul_done -> ball_in_other_half_did_foul [order 1] : [foul_loc_x < 6]
  throwing_foul_done -> ball_in_our_half [order 2] : [foul_loc_x > 6]
  in_play1 -> throwing_foul_done [order 1] : [foul_team_right == 1]
  in_play1 -> throwing_foul_not_done [order 3] : [foul_team_left == 1]
  throwing_foul_not_done -> in_play1 [order 1] : [foul_loc_x > 6 && after(2,sec)]
  init_pos_reached1 -> dont_stop_bot1 [order 2] : [stop == 0]
  ball_in_our_half -> init_pos_reached2 : [R_2_loc(1) <7.5 &&  R_2_loc(1) >7 && R_2_loc(2) <2.75 &&  R_2_loc(2) >2.25 && after(3,sec)]
  init_pos_reached1 -> stop_bot1 [order 1] : [stop == 1]
  dont_stop_bot1 -> in_play1 : [reset == 0 && after(3,sec)]
  stop_bot1 -> in_play1 : [bx > 5.6 || bx < 5.4 || by >4.1 || by<3.9]
  (default) -> in_play1
  init_pos_reached2 -> in_play1 : [[bx >foul_loc_x + 0.1  || bx < foul_loc_x - 0.1|| by >foul_loc_y + 0.1 || by<foul_loc_y - 0.1]]
  goal1 -> init_pos_reached1 : [R_2_loc(1) <7.5 &&  R_2_loc(1) >7 && R_2_loc(2) <2.75 &&  R_2_loc(2) >2.25 && after(3,sec)]
  in_play1 -> goal1 [order 2] : [reset == 1]
  data: R_2_loc input; bx input; by input; foul_loc_x input; foul_loc_y input; foul_team_left input; foul_team_right input; did_goal input; reset input; dest output; kick_UA output; stop local size=1; velocity_UA output

== stateflow chart Control_try_final_2020b/Team_2_Behaviour/T2_R3(Attacker 1)/Chart ==
  state ball_in_other_half_did_foul
    en:
    if (foul_loc_y>=7)
    dest = [foul_loc_x;foul_loc_y - 1;0];
    elseif(foul_loc_y<=1)
    dest = [foul_loc_x;foul_loc_y + 1;0];
    end
    kick_UA = 1;
    stop = 1;
  state reaching_foul
    du:
    velocity_UA = 1;
    dest = [bx;by;0];
  state throwing_foul_not_done
    du:
    dest = [foul_loc_x;foul_loc_y;0];
    kick_UA = 1;
  state throwing_foul_done
    du:
  state ball_in_our_half
    en:
    dest = [7.25;5.5;0];
    kick_UA = 1;
  state stop_bot
    du:
    velocity_UA = 1;
    dest = [bx;by;0];
  state dont_stop_bot
    du:
    velocity_UA = 1;
    dest = [bx;by;0];
  state in_play1
    du:
    dest = [bx;by;0];
    kick_UA = 0;
    stop = 0
    velocity_UA = 0;
  state goal1
    en:
    dest = [7.25;5.5;0];
    kick_UA = 1;
    if (did_goal == 1)
    stop = 1;
    else
    stop = 0;
    end
  state init_pos_reached1
    du:
  state init_pos
    du:
    velocity_UA = 1;
    dest = [bx;by;0];
  throwing_foul_not_done -> ball_in_our_half [order 2] : [foul_loc_x > 6]
  ball_in_other_half_did_foul -> reaching_foul : [R_2_loc(1) < foul_loc_x + 0.25 &&  R_2_loc(1) > foul_loc_x- 0.25 && R_2_loc(2) < foul_loc_y + 1.25 &&  R_2_loc(2) > foul_loc_y - 1.25 && after(3,sec)]
  throwing_foul_done -> ball_in_other_half_did_foul [order 1] : [foul_loc_x < 6]
  reaching_foul -> in_play1 : [bx >foul_loc_x + 0.1  || bx < foul_loc_x - 0.1|| by >foul_loc_y + 0.1 || by<foul_loc_y - 0.1]
  in_play1 -> throwing_foul_not_done [order 3] : [foul_team_left == 1 && after(2,sec)]
  throwing_foul_not_done -> in_play1 [order 1] : [foul_loc_x < 6 && after(20,sec) &&  bx < foul_loc_x + 0.1  && bx > foul_loc_x - 0.1 && by < foul_loc_y + 0.1  && by > foul_loc_y - 0.1]
  init_pos_reached1 -> dont_stop_bot [order 2] : [stop == 0]
  init_pos_reached1 -> stop_bot [order 1] : [stop == 1]
  throwing_foul_done -> ball_in_our_half [order 2] : [foul_loc_x > 6]
  in_play1 -> throwing_foul_done [order 1] : [foul_team_right == 1]
  ball_in_our_half -> init_pos : [R_2_loc(1) <7.5 &&  R_2_loc(1) >7 && R_2_loc(2) <5.75 &&  R_2_loc(2) >5.25 &&after(3,sec)]
  dont_stop_bot -> in_play1 : [reset == 0 && after(3,sec)]
  stop_bot -> in_play1 : [bx > 5.6 || bx < 5.4 || by >4.1 || by<3.9]
  (default) -> in_play1
  goal1 -> init_pos_reached1 : [R_2_loc(1) <7.5 &&  R_2_loc(1) >7 && R_2_loc(2) <5.75 &&  R_2_loc(2) >5.25 &&after(3,sec)]
  in_play1 -> goal1 [order 2] : [reset == 1]
  init_pos -> in_play1 : [[bx >foul_loc_x + 0.1  || bx < foul_loc_x - 0.1|| by >foul_loc_y + 0.1 || by<foul_loc_y - 0.1]]
  data: R_2_loc input; bx input; by input; foul_loc_x input; foul_loc_y input; foul_team_left input; foul_team_right input; did_goal input; reset input; dest output; kick_UA output; velocity_UA output; stop local

== stateflow chart Control_try_final_2020b/Team_2_Behaviour/T3_R4(Attacker 2)/Chart ==
  state ball_in_other_half_did_foul
    en:
    if (foul_loc_y>=7)
    dest = [foul_loc_x;foul_loc_y - 1;0];
    elseif(foul_loc_y<=1)
    dest = [foul_loc_x;foul_loc_y + 1;0];
    end
    kick_UA = 1;
    stop = 1;
  state reaching_foul
    du:
    velocity_UA = 1;
    dest = [bx;by;0];
  state throwing_foul_done
    du:
  state ball_in_our_half
    en:
    dest = [6;4;0];
    kick_UA = 1;
  state init_pos_reached2
    du:
    velocity_UA = 1;
    dest = [bx;by;0];
  state in_play1
    du:
    dest = [bx;by;0];
    kick_UA = 0;
    stop = 0
    velocity_UA = 0;
  state goal1
    en:
    dest = [6;4;0];
    kick_UA = 1;
    if (did_goal == 1)
    stop = 1;
    else
    stop = 0;
    end
  state reach_pos_CF
    en:
    velocity_UA = 1;
    dest = [bx;by;0];
  state Corner_foul_done
    en:
    dest = [3;2;0];
    kick_UA = 1;
  state init_pos_reached1
    du:
  state stop_bot
    du:
    velocity_UA = 1;
    dest = [bx;by;0];
  state dont_stop_bot
    du:
    velocity_UA = 1;
    dest = [bx;by;0];
  state corner_foul_not_done
    en:
    dest = [C_foul_loc_x;C_foul_loc_y;0];
    kick_UA = 1;
  ball_in_other_half_did_foul -> reaching_foul : [R_2_loc(1) < foul_loc_x + 1.25 &&  R_2_loc(1) > foul_loc_x- 1.25 && R_2_loc(2) < foul_loc_y + 1.25 &&  R_2_loc(2) > foul_loc_y - 1.25 && after(3,sec)]
  throwing_foul_done -> ball_in_other_half_did_foul [order 1] : [foul_loc_x < 6]
  reaching_foul -> in_play1 : [bx >foul_loc_x + 0.1  || bx < foul_loc_x - 0.1|| by >foul_loc_y + 0.1 || by<foul_loc_y - 0.1]
  throwing_foul_done -> ball_in_our_half [order 2] : [foul_loc_x > 6]
  in_play1 -> throwing_foul_done [order 1] : [foul_team_right == 1 || foul_team_left == 1 && after(1,sec)]
  ball_in_our_half -> init_pos_reached2 : [R_2_loc(1) <6.25 &&  R_2_loc(1) >5.75 && R_2_loc(2) <4.25 &&  R_2_loc(2) >3.75 && after(3,sec)]
  init_pos_reached2 -> in_play1 : [[bx >foul_loc_x + 0.1  || bx < foul_loc_x - 0.1|| by >foul_loc_y + 0.1 || by<foul_loc_y - 0.1]]
  (default) -> in_play1
  reach_pos_CF -> in_play1 : [(bx >1.6  || bx < 1.4 || by > 4.1 || by<3.9) && after(1,sec)]
  in_play1 -> goal1 [order 2] : [reset == 1]
  in_play1 -> Corner_foul_done [order 3] : [CFR == 1]
  in_play1 -> corner_foul_not_done [order 4] : [CFL == 1 && after(0.5,sec)]
  corner_foul_not_done -> in_play1 : [[R_2_loc(1) < C_foul_loc_x + 0.25 &&  R_2_loc(1) > C_foul_loc_x- 0.25 && R_2_loc(2) < C_foul_loc_y + 1.25 &&  R_2_loc(2) > C_foul_loc_y - 1.25 && after(3,sec)]]
  dont_stop_bot -> in_play1 : [reset == 0 && after(3,sec)]
  stop_bot -> in_play1 : [bx > 5.6 || bx < 5.4 || by >4.1 || by<3.9]
  goal1 -> init_pos_reached1 : [R_2_loc(1) <6.25 &&  R_2_loc(1) >5.75 && R_2_loc(2) <4.25 &&  R_2_loc(2) >3.75 && after(3,sec)]
  Corner_foul_done -> reach_pos_CF : [[(R_2_loc(1) <3.25 &&  R_2_loc(1) >2.75 && R_2_loc(2) <2.25 &&  R_2_loc(2) >1.75) ]]
  init_pos_reached1 -> stop_bot [order 1] : [stop == 1]
  init_pos_reached1 -> dont_stop_bot [order 2] : [stop == 0]
  data: R_2_loc input; bx input; by input; foul_loc_x input; foul_loc_y input; foul_team_left input; foul_team_right input; did_goal input; CFL input; CFR input; C_foul_loc_x input; C_foul_loc_y input; reset input; dest output; kick_UA output; stop local; velocity_UA output

== stateflow chart Control_try_final_2020b/Team_2_Behaviour/T2_R2(defender)/Team 1 Behaviour1/Chart1 ==
  state second_coordinate
    du:
    actual_angle = -pi +angle + angle_bot;
  state first_coordinate
    du:
    actual_angle = angle_bot - angle;
  state ffourth_coordinate
    du:
    actual_angle = -(2*pi) + angle + angle_bot
  state Third_coordinate
    du:
    actual_angle =-(pi) - angle + angle_bot;
  (default) -> first_coordinate
  first_coordinate -> second_coordinate [order 1] : [ Rx>Bx && Ry<By ]
  second_coordinate -> first_coordinate [order 1] : [ Rx<Bx && Ry<By]
  ffourth_coordinate -> second_coordinate [order 1] : [ Rx>Bx && Ry<By ]
  first_coordinate -> Third_coordinate [order 3] : [ Rx>Bx && Ry>By]
  second_coordinate -> Third_coordinate [order 3] : [ Rx>Bx && Ry>By ]
  Third_coordinate -> second_coordinate [order 1] : [ Rx>Bx && Ry<By ]
  second_coordinate -> ffourth_coordinate [order 2] : [ Rx<Bx && Ry>By ]
  Third_coordinate -> first_coordinate [order 2] : [ Rx<Bx && Ry<By ]
  ffourth_coordinate -> first_coordinate [order 2] : [ Rx<Bx && Ry<By ]
  first_coordinate -> ffourth_coordinate [order 2] : [ Rx<Bx && Ry>By ]
  Third_coordinate -> ffourth_coordinate [order 3] : [ Rx<Bx && Ry>By ]
  ffourth_coordinate -> Third_coordinate [order 3] : [ Rx>Bx && Ry>By]
  data: Bx input; By input; Rx input; Ry input; angle input; actual_angle output; angle_bot input

== stateflow chart Control_try_final_2020b/Team_2_Behaviour/T2_R2(defender)/Team 1 Behaviour1/Chart2 ==
  state go_to_ball
    du:
    kick = 0;
    pass_beh = 0;
    if(distance_to_ball < 0.25)
    pass_beh = pass_behaviour_controller(distance_to_goal,nearest_op,nearest_team);
    i = 0;
    else
    velocity = 0.44;
    end
  state avoid
    velocity = -(velocity);
  state pass
    du:
    velocity = 0;
    kick = 1;
  state shoot
    du:
    velocity = 0;
    kick = 1;
  state dribble
    du:
    velocity = 0;
    kick = 1;
  (default) -> go_to_ball
  go_to_ball -> avoid [order 1] : [nearest_rob < 0.3 && nearest_rob < 0 ]
  avoid -> go_to_ball : [nearest_rob > 1 ]
  go_to_ball -> pass [order 2] : [pass_beh == 1&& distance_to_ball < 0.25 ]
  dribble -> go_to_ball : [kick == 1]
  go_to_ball -> dribble [order 4] : [pass_beh == 2 && distance_to_ball < 0.25 ]
  pass -> go_to_ball : [kick == 1]
  go_to_ball -> shoot [order 3] : [pass_beh == 3 && distance_to_ball < 0.25 ]
  shoot -> go_to_ball : [kick == 1]
  data: distancetogoal function_input; nearest_oponent_distance function_input; nearest_team_player_distance function_input; pass_behaviour function_output; kick output =0; distance_to_ball input; velocity output; nearest_team input; nearest_op input; distance_to_goal input; pass_beh output =0; i local =1; nearest_rob input
  function pass_behaviour  = pass_behaviour_controller(distancetogoal,nearest_oponent_distance,nearest_team_player_distance):
    | function pass_behaviour  = pass_behaviour_controller(distancetogoal,nearest_oponent_distance,nearest_team_player_distance)
    | %PASS_BEHAVIOR Summary of this function goes here
    | %   Detailed explanation goes here
    | behaviourFuzzyFile= getFISCodeGenerationData('pass_behaviour.fis');
    | b = evalfis(behaviourFuzzyFile,[distancetogoal,nearest_oponent_distance,nearest_team_player_distance]);
    | 
    | if ( b<0.4 )
    | pass_behaviour=1;
    | elseif ( 0.4<=b && b<0.6 )
    | pass_behaviour=2;
    | else
    | pass_behaviour=3;
    | end
    | 
    | end

== stateflow chart Control_try_final_2020b/Team_2_Behaviour/T2_R2(defender)/Team 1 Behaviour1/Chart4 ==
  state stop
    du:
    w = 0;
    v=0.25 * velocity;
  state RCW
    du:
    w = -1*1;
    v=0;
  state RCCW
    du:
    w =1*1;
    v=0;
  (default) -> stop
  stop -> RCCW [order 2] : [after(1,sec) && DT > 0]
  stop -> RCW [order 1] : [after(1,sec) && DT < 0]
  RCW -> stop [order 1] : [DT<= 0.1 && DT>= -0.1]
  RCCW -> stop [order 1] : [DT<= 0.1 && DT>= -0.1]
  RCCW -> RCW [order 2] : [DT>0]
  RCW -> RCCW [order 2] : [DT<0]
  data: velocity input; v output; DT input; w output

== matlab function Control_try_final_2020b/Team_2_Behaviour/T2_R2(defender)/Team 1 Behaviour1/MATLAB Function ==
  data: F input; dF output; dis input; dT input
function dF = fcn(F,dis,dT)


F_x_max = max(abs(F(:,1))) ;
% F_y_max = max(abs(F(:,2))) ;

Fmax = sqrt((F_x_max^2)) ;

fc = sqrt(2*dis*dis*dT) ;

if fc <= Fmax
    dF = fc ;
else
    dF = Fmax ;
end

end

== matlab function Control_try_final_2020b/Team_2_Behaviour/T2_R2(defender)/Team 1 Behaviour1/MATLAB Function1 ==
  data: beh input; y output; goal input; team input; rob_loc input; rob_loc1 input; z output
function [y, z] = fcn(beh,goal,team,rob_loc,rob_loc1)
if (beh == 3)
    y = goal;
    z = [10,4];
elseif (beh == 2)
    y = 0.25;
    z = [10,4];
else
    y = team;
    z = [rob_loc1(1), rob_loc1(2)];
end

== stateflow chart Control_try_final_2020b/Team_1_behaviour/T1R2 (attacker 1)/Chart1 ==
  state reaching_foul
    du:
    velocity_UA = 1;
    dest = [bx;by;0];
  state ball_in_other_half_did_foul
    en:
    if (foul_loc_y>=7)
    dest = [foul_loc_x;foul_loc_y - 1;0];
    elseif(foul_loc_y<=1)
    dest = [foul_loc_x;foul_loc_y + 1;0];
    end
    kick_UA = 1;
    stop = 1;
  state throwing_foul
    du:
  state stop_bot1
    du:
    velocity_UA = 1;
    dest = [bx;by;0];
  state dont_stop_bot1
    du:
    velocity_UA = 1;
    dest = [bx;by;0];
  state ball_in_our_half
    en:
    dest = [3.25;2.5;0];
    kick_UA = 1;
  state init_pos_reached2
    du:
    velocity_UA = 1;
    dest = [bx;by;0];
  state in_play1
    du:
    dest = [bx;by;0];
    kick_UA = 0;
    stop = 0
    velocity_UA = 0;
  state goal1
    en:
    dest = [3.25;2.5;0];
    kick_UA = 1;
    if (did_goal == 1)
    stop = 1;
    else
    stop = 0;
    end
  state init_pos_reached1
    du:
  ball_in_other_half_did_foul -> reaching_foul : [R_2_loc(1) < foul_loc_x + 0.25 &&  R_2_loc(1) > foul_loc_x- 0.25 && R_2_loc(2) < foul_loc_y + 1.25 &&  R_2_loc(2) > foul_loc_y - 1.25 && after(3,sec)]
  reaching_foul -> in_play1 : [bx >foul_loc_x + 0.1  || bx < foul_loc_x - 0.1|| by >foul_loc_y + 0.1 || by<foul_loc_y - 0.1]
  init_pos_reached1 -> dont_stop_bot1 [order 2] : [stop == 0]
  throwing_foul -> ball_in_other_half_did_foul [order 1] : [foul_loc_x < 5.5]
  init_pos_reached1 -> stop_bot1 [order 1] : [stop == 1]
  throwing_foul -> ball_in_our_half [order 2] : [foul_loc_x > 5.5]
  in_play1 -> throwing_foul [order 1] : [foul_team_left == 1 || foul_team_right == 1]
  ball_in_our_half -> init_pos_reached2 : [R_2_loc(1) <3.5 &&  R_2_loc(1) >3 && R_2_loc(2) <2.75 &&  R_2_loc(2) >2.25 && after(3,sec)]
  dont_stop_bot1 -> in_play1 : [reset == 0 && after(3,sec)]
  stop_bot1 -> in_play1 : [bx > 5.6 || bx < 5.4 || by >4.1 || by<3.9]
  (default) -> in_play1
  goal1 -> init_pos_reached1 : [R_2_loc(1) <3.5 &&  R_2_loc(1) >3 && R_2_loc(2) <2.75 &&  R_2_loc(2) >2.25 && after(3,sec)]
  in_play1 -> goal1 [order 2] : [reset == 1]
  init_pos_reached2 -> in_play1 : [[bx >foul_loc_x + 0.1  || bx < foul_loc_x - 0.1|| by >foul_loc_y + 0.1 || by<foul_loc_y - 0.1]]
  data: R_2_loc input; bx input; by input; foul_team_right input; foul_team_left input; foul_loc_x input; foul_loc_y input; reset input; dest output; kick_UA output; velocity_UA output; did_goal input; stop local

== stateflow chart Control_try_final_2020b/Referee/Throwing ==
  state initilize
    en:
    foul_team_right = 0;
    foul_team_left = 0;
    throwin_foul_loc = [0;0]
  state out_filed
    en:
    if(bot_tag <5)
    foul_team_left = 1;
    foul_team_right = 0;
    else
    foul_team_left = 0;
    foul_team_right = 1;
    end
    throwin_foul_loc = [X;Y];
  state in_filed
    en:
    foul_team_right = 0;
    foul_team_left = 0;
    throwin_foul_loc = [0;0];
  (default) -> initilize
  initilize -> in_filed : [Y>=1 && Y<=7]
  in_filed -> out_filed : [Y>7 || Y<1]
  out_filed -> in_filed : [Y>=1 && Y<=7]
  data: foul_team_right output; X input; bot_tag input; Y input; foul_team_left output; throwin_foul_loc output

== matlab function Control_try_final_2020b/Enviornment/Ball_Dynamics1/MATLAB Function ==
  data: bot_tag input; pos input size=[1 3]; flag output
function flag  = fcn(bot_tag, pos)

X = pos(1) ;
Y = pos(2) ;
Z = pos(3) ;

% goal conditions
if X < 1 && Y > 2.7  && Y < 5.3 && Z < 1.2 
    flag = [1,5.5,4] ;
elseif fix(X) == 10 && Y > 2.7  && Y < 5.3 && Z <1.2
    flag = [1,5.5,4] ;
    
%corner conditions
elseif (X < 1 && (Y < 2.7 || Y > 5.3))
    if (bot_tag < 5)
        if (Y > 4)
            flag = [1,1,7] ;
        else
            flag = [1,1,1] ;
        end
    else
        flag = [1,1.5,4];
    end
elseif (X > 10 && (Y < 2.7 || Y > 5.3))
    if (bot_tag > 4)
        if (Y > 4)
             flag = [1,10,7] ;
        else
             flag = [1,10,1] ;
        end
    else
        flag = [1,5.5,4];
    end
% throwing conditions
elseif (Y < 1 || Y > 7)
     flag = [1,X,Y] ; 
% in game conditions
else
    flag = [0,5.5,4] ;
end

end

== stateflow chart Control_try_final_2020b/Team_1_behaviour/T1R2 (attacker 1)/Team 1 Behaviour1/Chart1 ==
  state second_coordinate
    du:
    actual_angle = -pi +angle + angle_bot;
  state first_coordinate
    du:
    actual_angle = angle_bot - angle;
  state ffourth_coordinate
    du:
    actual_angle = -(2*pi) + angle + angle_bot
  state Third_coordinate
    du:
    actual_angle =-(pi) - angle + angle_bot;
  (default) -> first_coordinate
  first_coordinate -> second_coordinate [order 1] : [ Rx>Bx && Ry<By ]
  second_coordinate -> first_coordinate [order 1] : [ Rx<Bx && Ry<By]
  ffourth_coordinate -> second_coordinate [order 1] : [ Rx>Bx && Ry<By ]
  first_coordinate -> Third_coordinate [order 3] : [ Rx>Bx && Ry>By]
  second_coordinate -> Third_coordinate [order 3] : [ Rx>Bx && Ry>By ]
  Third_coordinate -> second_coordinate [order 1] : [ Rx>Bx && Ry<By ]
  second_coordinate -> ffourth_coordinate [order 2] : [ Rx<Bx && Ry>By ]
  Third_coordinate -> first_coordinate [order 2] : [ Rx<Bx && Ry<By ]
  ffourth_coordinate -> first_coordinate [order 2] : [ Rx<Bx && Ry<By ]
  first_coordinate -> ffourth_coordinate [order 2] : [ Rx<Bx && Ry>By ]
  Third_coordinate -> ffourth_coordinate [order 3] : [ Rx<Bx && Ry>By ]
  ffourth_coordinate -> Third_coordinate [order 3] : [ Rx>Bx && Ry>By]
  data: Bx input; By input; Rx input; Ry input; angle input; actual_angle output; angle_bot input

== stateflow chart Control_try_final_2020b/Team_1_behaviour/T1R2 (attacker 1)/Team 1 Behaviour1/Chart2 ==
  state go_to_ball
    du:
    kick = 0;
    pass_beh = 0;
    if(distance_to_ball < 0.25)
    pass_beh = pass_behaviour_controller(distance_to_goal,nearest_op,nearest_team);
    i = 0;
    else
    velocity = 0.44;
    end
  state pass
    du:
    velocity = 0;
    kick = 1;
  state shoot
    du:
    velocity = 0;
    kick = 1;
  state dribble
    du:
    velocity = 0;
    kick = 1;
  (default) -> go_to_ball
  go_to_ball -> pass [order 1] : [pass_beh == 1&& distance_to_ball < 0.25 ]
  dribble -> go_to_ball : [kick == 1]
  go_to_ball -> dribble [order 3] : [pass_beh == 2 && distance_to_ball < 0.25 ]
  pass -> go_to_ball : [kick == 1]
  go_to_ball -> shoot [order 2] : [pass_beh == 3 && distance_to_ball < 0.25 ]
  shoot -> go_to_ball : [kick == 1]
  data: distancetogoal function_input; nearest_oponent_distance function_input; nearest_team_player_distance function_input; pass_behaviour function_output; kick output =0; distance_to_ball input; velocity output; nearest_team input; nearest_op input; distance_to_goal input; pass_beh output =0; i local =1
  function pass_behaviour  = pass_behaviour_controller(distancetogoal,nearest_oponent_distance,nearest_team_player_distance):
    | function pass_behaviour  = pass_behaviour_controller(distancetogoal,nearest_oponent_distance,nearest_team_player_distance)
    | %PASS_BEHAVIOR Summary of this function goes here
    | %   Detailed explanation goes here
    | behaviourFuzzyFile= getFISCodeGenerationData('pass_behaviour.fis');
    | b = evalfis(behaviourFuzzyFile,[distancetogoal,nearest_oponent_distance,nearest_team_player_distance]);
    | 
    | if ( b<0.4 )
    | pass_behaviour=1;
    | elseif ( 0.4<=b && b<0.6 )
    | pass_behaviour=2;
    | else
    | pass_behaviour=3;
    | end
    | 
    | end

== stateflow chart Control_try_final_2020b/Team_1_behaviour/T1R2 (attacker 1)/Team 1 Behaviour1/Chart4 ==
  state stop
    du:
    w = 0;
    v=0.25 * velocity;
  state RCW
    du:
    w = -1*1;
    v=0;
  state RCCW
    du:
    w =1*1;
    v=0;
  (default) -> stop
  stop -> RCCW [order 2] : [after(1,sec) && DT > 0]
  stop -> RCW [order 1] : [after(1,sec) && DT < 0]
  RCW -> stop [order 1] : [DT<= 0.1 && DT>= -0.1]
  RCCW -> stop [order 1] : [DT<= 0.1 && DT>= -0.1]
  RCCW -> RCW [order 2] : [DT>0]
  RCW -> RCCW [order 2] : [DT<0]
  data: velocity input; v output; DT input; w output

== matlab function Control_try_final_2020b/Team_1_behaviour/T1R2 (attacker 1)/Team 1 Behaviour1/MATLAB Function ==
  data: F input; dF output; dis input; dT input
function dF = fcn(F,dis,dT)


F_x_max = max(abs(F(:,1))) ;
% F_y_max = max(abs(F(:,2))) ;

Fmax = sqrt((F_x_max^2)) ;

fc = sqrt(2*dis*dis*dT) ;

if fc <= Fmax
    dF = fc ;
else
    dF = Fmax ;
end

end

== matlab function Control_try_final_2020b/Team_1_behaviour/T1R2 (attacker 1)/Team 1 Behaviour1/MATLAB Function1 ==
  data: beh input; y output; goal input; team input; rob_loc input; rob_loc1 input; z output
function [y, z] = fcn(beh,goal,team,rob_loc,rob_loc1)
if (beh == 3)
    y = goal;
    z = [10,4];
elseif (beh == 2)
    y = 0.25;
    z = [10,4];
else
    y = team;
    z = [rob_loc1(1), rob_loc1(2)];
end

== matlab function Control_try_final_2020b/Team_1_behaviour/T1R3 (Defender 2)/Team 1 Behaviour1/MATLAB Function2 ==
  data: u input; y output; r3 input; r4 input
function y = fcn(u , r3, r4)
if u == 2
   y = [r3(1), r3(2)];
else
    y = [r4(1) , r4(2)];
end

== stateflow chart Control_try_final_2020b/Team_1_behaviour/T1R2 (attacker 1)/Team 1 Behaviour1/kick_direction1/Chart1 ==
  state x_pos
    du:
    Vx = 1
  state x_neg
    du:
    Vx = -1
  (default) -> x_pos
  x_pos -> x_neg : [x > 0]
  x_neg -> x_pos : [x<1]
  data: Vx output; x input

== stateflow chart Control_try_final_2020b/Team_2_Behaviour/T2_R3(Attacker 1)/Team 1 Behaviour1/Chart5 ==
  state stop
    du:
    w = 0;
    v=0.25 * velocity;
  state RCW
    du:
    w = -1*1;
    v=0;
  state RCCW
    du:
    w =1*1;
    v=0;
  (default) -> stop
  stop -> RCCW [order 2] : [after(1,sec) && DT > 0]
  stop -> RCW [order 1] : [after(1,sec) && DT < 0]
  RCW -> stop [order 1] : [DT<= 0.1 && DT>= -0.1]
  RCCW -> stop [order 1] : [DT<= 0.1 && DT>= -0.1]
  RCCW -> RCW [order 2] : [DT>0]
  RCW -> RCCW [order 2] : [DT<0]
  data: velocity input; v output; DT input; w output
